simulink model "test_com_SensorFusion_e8"  (R2017a)
settings: Solver=FixedStepAuto  StartTime=250  StopTime=450  RelTol=1e-3
undefined symbols (not defined in the file or in its folder): DiscIntNeverNeededParam, GearRatio
settings Model: DataDictionary=controller_dict.sldd  SnapshotInterval=100  Creator=daniel  LastModifiedBy=gt_testing
settings DataIOCC: ExternalInput=VD_Gyro_Front_Accel_X, VD_Gyro_Front_Accel_Y, VD_Gyro_Front_Accel_Z,VD_Gyro_Front_ARate_X, VD_Gyro_Front_ARate_Y, VD_Gyro_Front_ARate_Z, VD_Gyro_Front_Comp_X, VD_Gyro_Front_Comp_Y, VD_Gyro_Front_Comp_Z, VD_Gyro_Front_Temp, VD_Gyro_Rear_Accel_X, VD_Gyro_Rear_Accel_Y, VD_Gyro_Rear_Accel_Z, VD_Gyro_Rear_ARate_X, VD_Gyro_Rear_ARate_Y, VD_Gyro_Rear_ARate_Z, VD_Gyro_Rear_Comp_X, VD_Gyro_Rear_Comp_Y, VD_Gyro_Rear_Comp_Z, VD_Gyro_Rear_Temp, VD_V2O_SpeedLongitudinal, VD_V2O_SpeedLateral, PT_MotorSpeed_FL, PT_MotorSpeed_FR, PT_MotorSpeed_RL, PT_MotorSpeed_RR  LimitDataPoints=on  LoadExternalInput=on  SaveFormat=Array  SaveOutput=off  SignalLogging=off  DSMLogging=off  SaveTime=off
settings OptimizationCC: DefaultParameterBehavior=Inlined  UseDivisionForNetSlopeComputation=on  StateBitsets=on  DataBitsets=on  LifeSpan=1
settings DebuggingCC: SolverPrmCheckMsg=warning  ParameterPrecisionLossMsg=none  AllowSymbolicDim=off  SFUnexpectedBacktrackingDiag=warning  SFNoUnconditionalDefaultTransitionDiag=warning  SFExecutionAtInitializationDiag=none
settings HardwareCC: ProdBitPerPointer=32  ProdBitPerSizeT=32  ProdBitPerPtrDiffT=32  ProdLargestAtomicInteger=Long  ProdLargestAtomicFloat=Double  ProdWordSize=32  ProdHWDeviceType=Texas Instruments->TMS570 Cortex-R4
settings ModelReferenceCC: PropagateSignalLabelsOutOfModel=off
settings SFSimCC: SimBuildMode=sf_nonincremental_build  MATLABDynamicMemAlloc=off
settings RTWCC: SystemTargetFile=ert.tlc  GenCodeOnly=on  TemplateMakefile=ert_default_tmf  Description=Embedded Coder  GenerateReport=on  BuildConfiguration=Faster Runs  IncludeHyperlinkInReport=on  LaunchReport=on  GenerateTraceReport=on
settings CodeAppCC: IgnoreCustomStorageClasses=off  SFDataObjDesc=on
settings ERTTargetCC: MultiwordLength=2048  GenerateSampleERTMain=on  InlinedParameterPlacement=NonHierarchical  ERTCustomFileTemplate=example_file_process.tlc  ConvertIfToSwitch=off  SuppressUnreachableDefaultCases=off
settings ConfigComp: CovMetricSettings=dw  CovHtmlReporting=on  CovSaveCumulativeToWorkspaceVar=on  CovSaveSingleToWorkspaceVar=on  CovExternalEMLEnable=off  CovSFcnEnable=off
settings ConfigurationSet: Description=SimMechanics 2G

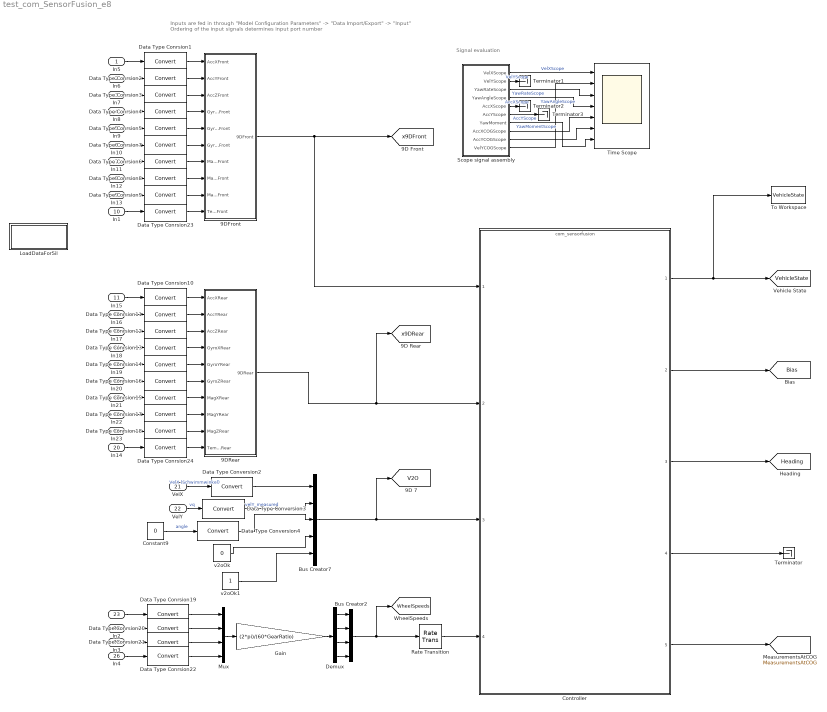
== system test_com_SensorFusion_e8 ==
  note: Signal evaluation
  note: Inputs are fed in through "Model Configuration Parameters" -> "Data Import/Export" -> "Input"
      | Ordering of the input signals determines input port number
  In5 : Inport  OutDataTypeStr=single  LockScale=on
  In6 : Inport  Port=2
  In7 : Inport  Port=3
  In8 : Inport  Port=4
  In9 : Inport  Port=5
  In10 : Inport  Port=6
  In11 : Inport  Port=7
  In12 : Inport  Port=8
  In13 : Inport  Port=9
  In1 : Inport  Port=10
  In15 : Inport  Port=11
  In16 : Inport  Port=12
  In17 : Inport  Port=13
  In18 : Inport  Port=14
  In19 : Inport  Port=15
  In20 : Inport  Port=16
  In21 : Inport  Port=17
  In22 : Inport  Port=18
  In23 : Inport  Port=19
  In14 : Inport  Port=20
  VelX : Inport  Port=21
  VelY : Inport  Port=22
  " " : Inport  Port=23
  In2 : Inport  Port=24
  In3 : Inport  Port=25
  In4 : Inport  Port=26
  9DFront : Subsystem
  9DRear : Subsystem
  Bus Creator2 : BusCreator  Inputs=4  OutDataTypeStr=Bus: control_WheelSpeed
      settings: InheritFromInputs=off
  Bus Creator7 : BusCreator  Inputs=5  OutDataTypeStr=Bus: control_velocity
      settings: InheritFromInputs=off
  Constant9 : Constant  Value=0  OutDataTypeStr=Inherit: Inherit via back propagation
  Controller : ModelReference  ModelNameDialog=com_sensorfusion.slx  SimulationMode=Normal  ModelReferenceVersion=1.1521
  Data Type Conrsion{1..24} (24 alike) : DataTypeConversion
  Data Type Conversion2 : DataTypeConversion
  Data Type Conversion3 : DataTypeConversion
  Data Type Conversion4 : DataTypeConversion
  Demux : Demux
  Gain : Gain  Gain=(2*pi)/(60*GearRatio)
  LoadDataForSil : Subsystem
      settings: OpenFcn=LoadDataForSil
  Mux : Mux
  Rate Transition : RateTransition  OutPortSampleTime=0.002
  Scope signal assembly : Subsystem
  Terminator{,1..3} (4 alike) : Terminator
  Time Scope : Scope  NumInputPorts=7
  To Workspace : ToWorkspace  VariableName=VehicleState  SaveFormat=Timeseries  SampleTime=-1
  v2oOk : Constant  Value=0  OutDataTypeStr=boolean
  v2oOk1 : Constant  OutDataTypeStr=boolean
  tag scope: Bias=global, Heading=global, MeasurementsAtCOG=global, V2O=global, VehicleState=global, WheelSpeeds=global, x9DFront=global, x9DRear=global
  wires:
  Bus Creator7/1 -> [V2O], Controller/3
  VelY/1 -> Data Type Conversion3/1  "vq"
  Constant9/1 -> Data Type Conversion4/1  "angle"
  Demux/1 -> Bus Creator2/1
  Demux/2 -> Bus Creator2/2
  Demux/3 -> Bus Creator2/3
  Gain/1 -> Demux/1
  Mux/1 -> Gain/1
  " "/1 -> Data Type Conrsion19/1
  In2/1 -> Data Type Conrsion20/1
  In3/1 -> Data Type Conrsion21/1
  In4/1 -> Data Type Conrsion22/1
  VelX/1 -> Data Type Conversion2/1  "VelX (Schwimmwinkel)"
  Data Type Conversion3/1 -> Bus Creator7/2  "velY_measured"
  Demux/4 -> Bus Creator2/4
  In5/1 -> Data Type Conrsion1/1
  In6/1 -> Data Type Conrsion2/1
  In7/1 -> Data Type Conrsion3/1
  In8/1 -> Data Type Conrsion4/1
  In9/1 -> Data Type Conrsion5/1
  In10/1 -> Data Type Conrsion7/1
  In11/1 -> Data Type Conrsion6/1
  In12/1 -> Data Type Conrsion8/1
  In13/1 -> Data Type Conrsion9/1
  Data Type Conrsion23/1 -> 9DFront/10(Temp9DFront)
  Controller/1 -> To Workspace/1, [VehicleState]
  Controller/2 -> [Bias]
  Controller/3 -> [Heading]
  Scope signal assembly/1(VelXScope) -> Time Scope/1  "VelXScope"
  Scope signal assembly/3(YawRateScope) -> Time Scope/3  "YawRateScope"
  Scope signal assembly/4(YawAngleScope) -> Time Scope/4  "YawAngleScope"
  Controller/4 -> Terminator/1
  Bus Creator2/1 -> [WheelSpeeds], Rate Transition/1
  Scope signal assembly/7(YawMoment) -> Time Scope/7  "YawMomentScope"
  Controller/5 -> [MeasurementsAtCOG]
  Scope signal assembly/8(AccXCOGScope) -> Time Scope/5
  Scope signal assembly/9(AccYCOGScope) -> Time Scope/6
  Scope signal assembly/10(VelYCOGScope) -> Time Scope/2
  Scope signal assembly/2(VelYScope) -> Terminator1/1  "VelYScope"
  Scope signal assembly/5(AccXScope) -> Terminator2/1  "AccXScope"
  Scope signal assembly/6(AccYScope) -> Terminator3/1  "AccYScope"
  v2oOk/1 -> Bus Creator7/4
  v2oOk1/1 -> Bus Creator7/5
  Rate Transition/1 -> Controller/4
  9DFront/1(9DFront) -> [x9DFront], Controller/1
  9DRear/1(9DRear) -> [x9DRear], Controller/2
  Data Type Conversion2/1 -> Bus Creator7/1
  Data Type Conversion4/1 -> Bus Creator7/3
  Data Type Conrsion1/1 -> 9DFront/1(AccXFront)
  Data Type Conrsion2/1 -> 9DFront/2(AccYFront)
  Data Type Conrsion3/1 -> 9DFront/3(AccZFront)
  Data Type Conrsion4/1 -> 9DFront/4(GyroXFront)
  Data Type Conrsion5/1 -> 9DFront/5(GyroYFront)
  Data Type Conrsion7/1 -> 9DFront/6(GyroZFront)
  Data Type Conrsion6/1 -> 9DFront/7(MagXFront)
  Data Type Conrsion8/1 -> 9DFront/8(MagYFront)
  Data Type Conrsion9/1 -> 9DFront/9(MagZFront)
  In22/1 -> Data Type Conrsion17/1
  In21/1 -> Data Type Conrsion15/1
  In20/1 -> Data Type Conrsion16/1
  In19/1 -> Data Type Conrsion14/1
  In18/1 -> Data Type Conrsion13/1
  In17/1 -> Data Type Conrsion12/1
  In16/1 -> Data Type Conrsion11/1
  In15/1 -> Data Type Conrsion10/1
  In23/1 -> Data Type Conrsion18/1
  Data Type Conrsion10/1 -> 9DRear/1(AccXRear)
  Data Type Conrsion11/1 -> 9DRear/2(AccYRear)
  Data Type Conrsion12/1 -> 9DRear/3(AccZRear)
  Data Type Conrsion13/1 -> 9DRear/4(GyroXRear)
  Data Type Conrsion14/1 -> 9DRear/5(GyroYRear)
  Data Type Conrsion16/1 -> 9DRear/6(GyroZRear)
  Data Type Conrsion15/1 -> 9DRear/7(MagXRear)
  Data Type Conrsion17/1 -> 9DRear/8(MagYRear)
  Data Type Conrsion18/1 -> 9DRear/9(MagZRear)
  Data Type Conrsion19/1 -> Mux/1
  Data Type Conrsion20/1 -> Mux/2
  Data Type Conrsion21/1 -> Mux/3
  Data Type Conrsion22/1 -> Mux/4
  In1/1 -> Data Type Conrsion23/1
  In14/1 -> Data Type Conrsion24/1
  Data Type Conrsion24/1 -> 9DRear/10(Temp9DRear)

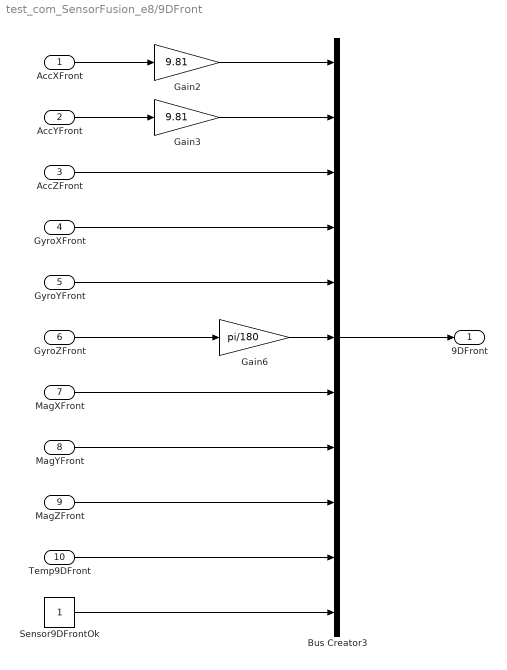
== system test_com_SensorFusion_e8/9DFront ==
  AccXFront : Inport
  AccYFront : Inport  Port=2
  AccZFront : Inport  Port=3
  GyroXFront : Inport  Port=4
  GyroYFront : Inport  Port=5
  GyroZFront : Inport  Port=6
  MagXFront : Inport  Port=7
  MagYFront : Inport  Port=8
  MagZFront : Inport  Port=9
  Temp9DFront : Inport  Port=10
  Bus Creator3 : BusCreator  Inputs=11  OutDataTypeStr=Bus: control_9D_Full_float
      settings: InheritFromInputs=off
  Gain2 : Gain  Gain=9.81
  Gain3 : Gain  Gain=9.81
  Gain6 : Gain  Gain=pi/180
  Sensor9DFrontOk : Constant  OutDataTypeStr=boolean
  9DFront : Outport
  wires:
  AccXFront/1 -> Gain2/1
  Temp9DFront/1 -> Bus Creator3/10
  GyroZFront/1 -> Gain6/1
  AccZFront/1 -> Bus Creator3/3
  AccYFront/1 -> Gain3/1
  GyroYFront/1 -> Bus Creator3/5
  MagZFront/1 -> Bus Creator3/9
  Gain2/1 -> Bus Creator3/1
  Bus Creator3/1 -> 9DFront/1
  MagYFront/1 -> Bus Creator3/8
  MagXFront/1 -> Bus Creator3/7
  Gain6/1 -> Bus Creator3/6
  GyroXFront/1 -> Bus Creator3/4
  Gain3/1 -> Bus Creator3/2
  Sensor9DFrontOk/1 -> Bus Creator3/11

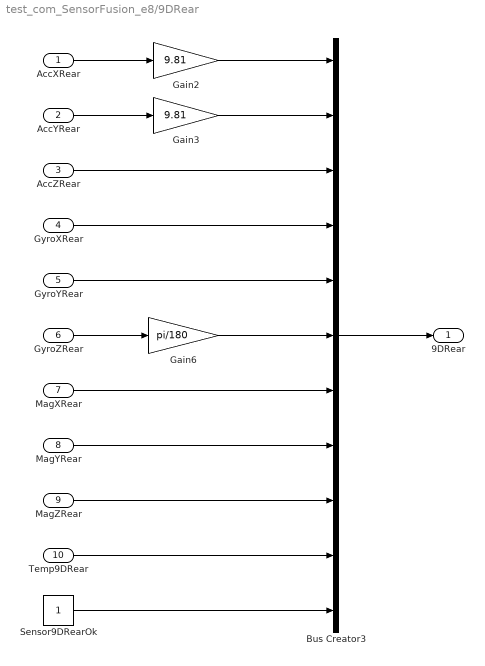
== system test_com_SensorFusion_e8/9DRear ==
  AccXRear : Inport
  AccYRear : Inport  Port=2
  AccZRear : Inport  Port=3
  GyroXRear : Inport  Port=4
  GyroYRear : Inport  Port=5
  GyroZRear : Inport  Port=6
  MagXRear : Inport  Port=7
  MagYRear : Inport  Port=8
  MagZRear : Inport  Port=9
  Temp9DRear : Inport  Port=10
  Bus Creator3 : BusCreator  Inputs=11  OutDataTypeStr=Bus: control_9D_Full_float
      settings: InheritFromInputs=off
  Gain2 : Gain  Gain=9.81
  Gain3 : Gain  Gain=9.81
  Gain6 : Gain  Gain=pi/180
  Sensor9DRearOk : Constant  OutDataTypeStr=boolean
  9DRear : Outport
  wires:
  GyroXRear/1 -> Bus Creator3/4
  MagXRear/1 -> Bus Creator3/7
  MagYRear/1 -> Bus Creator3/8
  Bus Creator3/1 -> 9DRear/1
  Gain3/1 -> Bus Creator3/2
  Gain2/1 -> Bus Creator3/1
  MagZRear/1 -> Bus Creator3/9
  GyroYRear/1 -> Bus Creator3/5
  AccYRear/1 -> Gain3/1
  AccZRear/1 -> Bus Creator3/3
  GyroZRear/1 -> Gain6/1
  Temp9DRear/1 -> Bus Creator3/10
  AccXRear/1 -> Gain2/1
  Sensor9DRearOk/1 -> Bus Creator3/11
  Gain6/1 -> Bus Creator3/6

== system test_com_SensorFusion_e8/LoadDataForSil ==

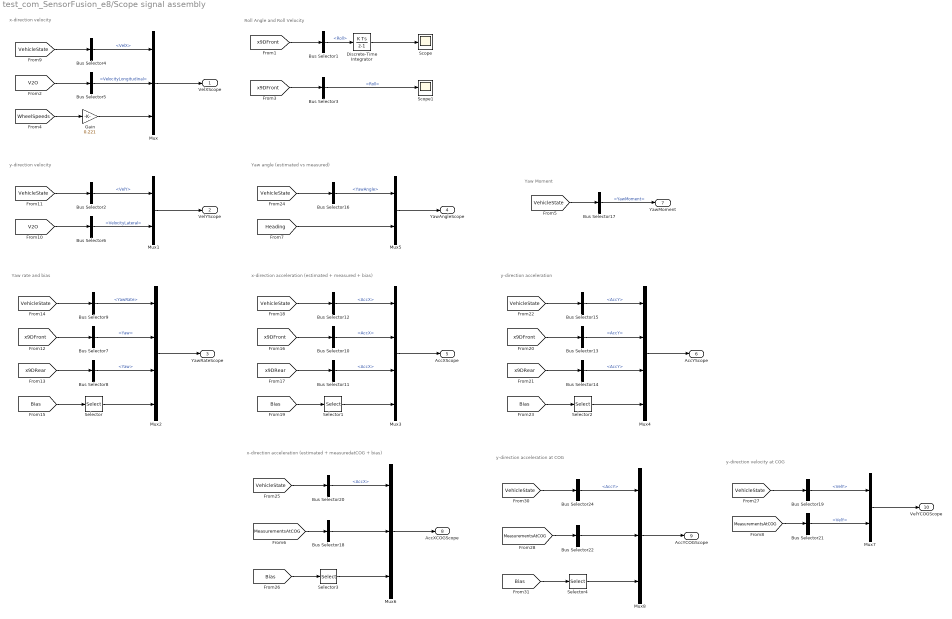
== system test_com_SensorFusion_e8/Scope signal assembly ==
  note: Yaw Moment
  note: Roll Angle and Roll Velocity
  note: Yaw angle (estimated vs measured)
  note: x-direction acceleration (estimated + measured + bias)
  note: Yaw rate and bias
  note: y-direction velocity
  note: x-direction velocity
  note: y-direction acceleration
  note: x-direction acceleration (estimated + measuredatCOG + bias)
  note: y-direction velocity at COG
  note: y-direction acceleration at COG
  Bus Selector1 : BusSelector  OutputSignals=Roll
  Bus Selector{10..12,20} (4 alike) : BusSelector  OutputSignals=AccX
  Bus Selector{13..15,24} (4 alike) : BusSelector  OutputSignals=AccY
  Bus Selector16 : BusSelector  OutputSignals=YawAngle
  Bus Selector17 : BusSelector  OutputSignals=YawMoment
  Bus Selector18 : BusSelector  OutputSignals=AccXFront,AccXRear  OutputAsBus=on
  Bus Selector19 : BusSelector  OutputSignals=VelY
  Bus Selector2 : BusSelector  OutputSignals=VelY
  Bus Selector21 : BusSelector  OutputSignals=VelY
  Bus Selector22 : BusSelector  OutputSignals=AccYFront,AccYRear  OutputAsBus=on
  Bus Selector3 : BusSelector  OutputSignals=Roll
  Bus Selector4 : BusSelector  OutputSignals=VelX
  Bus Selector5 : BusSelector  OutputSignals=VelocityLongitudinal
  Bus Selector6 : BusSelector  OutputSignals=VelocityLateral
  Bus Selector7 : BusSelector  OutputSignals=Yaw
  Bus Selector8 : BusSelector  OutputSignals=Yaw
  Bus Selector9 : BusSelector  OutputSignals=YawRate
  Discrete-Time Integrator : DiscreteIntegrator  InitialConditionSetting=State (most efficient)  SampleTime=-1  ICPrevOutput=DiscIntNeverNeededParam  ICPrevScaledInput=DiscIntNeverNeededParam
  Gain : Gain  Gain=0.221
  Mux : Mux  Inputs=3
  Mux1 : Mux  Inputs=2
  Mux2 : Mux
  Mux3 : Mux
  Mux4 : Mux
  Mux5 : Mux  Inputs=2
  Mux6 : Mux  Inputs=3
  Mux7 : Mux  Inputs=2
  Mux8 : Mux  Inputs=3
  Scope : Scope
  Scope1 : Scope
  Selector : Selector  InputPortWidth=6  IndexOptions=Index vector (dialog)  Indices=[5 6]  OutputSizes=1
  Selector1 : Selector  InputPortWidth=6  IndexOptions=Index vector (dialog)  Indices=[1 3]  OutputSizes=1
  Selector2 : Selector  InputPortWidth=6  IndexOptions=Index vector (dialog)  Indices=[2 4]  OutputSizes=1
  Selector3 : Selector  InputPortWidth=6  IndexOptions=Index vector (dialog)  Indices=[1 3]  OutputSizes=1
  Selector4 : Selector  InputPortWidth=6  IndexOptions=Index vector (dialog)  Indices=[2 4]  OutputSizes=1
  VelXScope : Outport
  VelYScope : Outport  Port=2
  YawRateScope : Outport  Port=3
  YawAngleScope : Outport  Port=4
  AccXScope : Outport  Port=5
  AccYScope : Outport  Port=6
  YawMoment : Outport  Port=7
  AccXCOGScope : Outport  Port=8
  AccYCOGScope : Outport  Port=9
  VelYCOGScope : Outport  Port=10
  wires:
  [WheelSpeeds] -> Gain/1
  [V2O] -> Bus Selector5/1
  [VehicleState] -> Bus Selector4/1
  Bus Selector4/1 -> Mux/1  "<VelX>"
  Bus Selector5/1 -> Mux/2  "<VelocityLongitudinal>"
  Mux/1 -> VelXScope/1
  [V2O] -> Bus Selector6/1
  [VehicleState] -> Bus Selector2/1
  Bus Selector2/1 -> Mux1/1  "<VelY>"
  Bus Selector6/1 -> Mux1/2  "<VelocityLateral>"
  Mux1/1 -> VelYScope/1
  [x9DFront] -> Bus Selector7/1
  [x9DRear] -> Bus Selector8/1
  [VehicleState] -> Bus Selector9/1
  [Bias] -> Selector/1
  Bus Selector9/1 -> Mux2/1  "<YawRate>"
  Bus Selector7/1 -> Mux2/2  "<Yaw>"
  Bus Selector8/1 -> Mux2/3  "<Yaw>"
  Selector/1 -> Mux2/4
  Mux2/1 -> YawRateScope/1
  [x9DFront] -> Bus Selector10/1
  [x9DRear] -> Bus Selector11/1
  [VehicleState] -> Bus Selector12/1
  [Bias] -> Selector1/1
  Bus Selector12/1 -> Mux3/1  "<AccX>"
  Bus Selector10/1 -> Mux3/2  "<AccX>"
  Bus Selector11/1 -> Mux3/3  "<AccX>"
  Selector1/1 -> Mux3/4
  Mux3/1 -> AccXScope/1
  [x9DFront] -> Bus Selector13/1
  [x9DRear] -> Bus Selector14/1
  [VehicleState] -> Bus Selector15/1
  [Bias] -> Selector2/1
  Bus Selector15/1 -> Mux4/1  "<AccY>"
  Bus Selector13/1 -> Mux4/2  "<AccY>"
  Bus Selector14/1 -> Mux4/3  "<AccY>"
  Selector2/1 -> Mux4/4
  Mux4/1 -> AccYScope/1
  [VehicleState] -> Bus Selector16/1
  Bus Selector16/1 -> Mux5/1  "<YawAngle>"
  [Heading] -> Mux5/2
  Mux5/1 -> YawAngleScope/1
  [x9DFront] -> Bus Selector1/1
  Bus Selector1/1 -> Discrete-Time Integrator/1  "<Roll>"
  Discrete-Time Integrator/1 -> Scope/1
  [x9DFront] -> Bus Selector3/1
  Bus Selector3/1 -> Scope1/1  "<Roll>"
  Gain/1 -> Mux/3
  [VehicleState] -> Bus Selector17/1
  Bus Selector17/1 -> YawMoment/1  "<YawMoment>"
  Bus Selector18/1 -> Mux6/2
  [VehicleState] -> Bus Selector20/1
  Bus Selector20/1 -> Mux6/1  "<AccX>"
  Mux6/1 -> AccXCOGScope/1
  [Bias] -> Selector3/1
  [MeasurementsAtCOG] -> Bus Selector18/1
  Selector3/1 -> Mux6/3
  Mux7/1 -> VelYCOGScope/1
  [VehicleState] -> Bus Selector19/1
  Bus Selector19/1 -> Mux7/1  "<VelY>"
  [MeasurementsAtCOG] -> Bus Selector21/1
  Bus Selector21/1 -> Mux7/2  "<VelY>"
  Mux8/1 -> AccYCOGScope/1
  Selector4/1 -> Mux8/3
  Bus Selector24/1 -> Mux8/1  "<AccY>"
  Bus Selector22/1 -> Mux8/2
  [Bias] -> Selector4/1
  [MeasurementsAtCOG] -> Bus Selector22/1
  [VehicleState] -> Bus Selector24/1
